simulink model "heave_tracking"  (R2020a)
settings: Solver=VariableStepAuto  StartTime=0.0  StopTime=50  FixedStep=0.001  MaxStep=0.001  RelTol=1e-3  EnableMultiTasking=on
values from neighbouring files (symbols this model uses):
  aw = -728/(1862.87+3660)    (= -0.131815523451)    [heave_tracking_1.m]
  bw = 1/(1862.87+3660)    (= 0.000181065279465)    [heave_tracking_1.m]
  F = [K eye(mm)]*inv(TT)    [heave_tracking_1.m]
  Z_w_bar = -1821/(1862.87+3660)    (= -0.329719873906)    [heave_tracking_1.m]
settings Model: Creator=xiaoran  LastModifiedBy=xiaoran
settings DataIOCC: LimitDataPoints=on  SaveFormat=Array  ReturnWorkspaceOutputs=off
settings OptimizationCC: LifeSpan=inf
settings DebuggingCC: UnderspecifiedInitializationDetection=Classic  MergeDetectMultiDrivingBlocksExec=none  SolverPrmCheckMsg=warning  StateNameClashWarn=warning  SFUnexpectedBacktrackingDiag=warning  SFNoUnconditionalDefaultTransitionDiag=warning  SFExecutionAtInitializationDiag=none  ArithmeticOperatorsInVariantConditions=warning
settings HardwareCC: ProdBitPerPointer=32  ProdBitPerSizeT=32  ProdBitPerPtrDiffT=32  ProdLargestAtomicFloat=None  ProdIntDivRoundTo=Undefined  ProdEndianess=Unspecified  ProdWordSize=32  ProdHWDeviceType=32-bit Generic
settings ModelReferenceCC: PropagateSignalLabelsOutOfModel=off
settings SFSimCC: SimUseLocalCustomCode=off  CustomCodeUndefinedFunction=UseInterfaceOnly
settings RTWCC: RTWUseLocalCustomCode=off
settings CodeAppCC: StateflowObjectComments=on
settings GRTTargetCC: TargetLangStandard=C89/C90 (ANSI)
settings ConfigComp: CovMetricSettings=dw  CovHtmlReporting=on  CovSaveCumulativeToWorkspaceVar=on  CovSaveSingleToWorkspaceVar=on  CovExternalEMLEnable=off

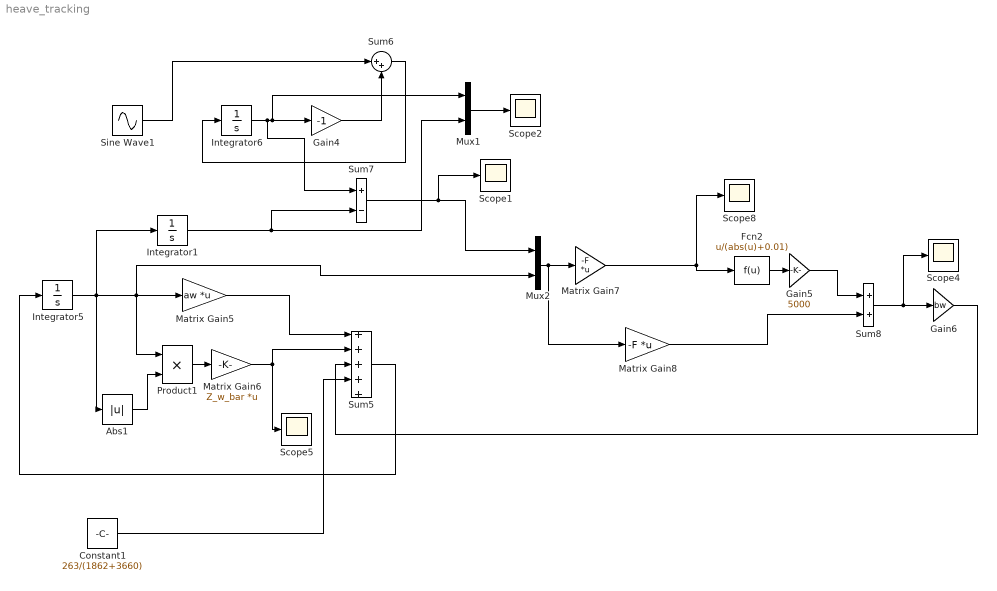
== system heave_tracking ==
  Abs1 : Abs
  Constant1 : Constant  Value=263/(1862+3660)
  Fcn2 : Fcn  Expr=u/(abs(u)+0.01)
  Gain4 : Gain  Gain=-1
  Gain5 : Gain  Gain=5000  SaturateOnIntegerOverflow=on  OutDataTypeStr=Inherit: Same as input  ParamDataTypeStr=Inherit: Same as input
  Gain6 : Gain  Gain=bw  SaturateOnIntegerOverflow=on  OutDataTypeStr=Inherit: Same as input  ParamDataTypeStr=Inherit: Same as input
  Integrator1 : Integrator  InitialCondition=0.1
  Integrator5 : Integrator  InitialCondition=0.1
  Integrator6 : Integrator  InitialCondition=.1
  Matrix Gain5 : Gain  Gain=aw  Multiplication=Matrix(K*u)  SaturateOnIntegerOverflow=on  OutDataTypeStr=Inherit: Same as input  ParamDataTypeStr=Inherit: Same as input
  Matrix Gain6 : Gain  Gain=Z_w_bar  Multiplication=Matrix(K*u)  SaturateOnIntegerOverflow=on  OutDataTypeStr=Inherit: Same as input  ParamDataTypeStr=Inherit: Same as input
  Matrix Gain7 : Gain  Gain=-F  Multiplication=Matrix(K*u)  SaturateOnIntegerOverflow=on  OutDataTypeStr=Inherit: Same as input  ParamDataTypeStr=Inherit: Same as input
  Matrix Gain8 : Gain  Gain=-F  Multiplication=Matrix(K*u)  SaturateOnIntegerOverflow=on  OutDataTypeStr=Inherit: Same as input  ParamDataTypeStr=Inherit: Same as input
  Mux1 : Mux  Inputs=2
  Mux2 : Mux  Inputs=2
  Product1 : Product
  Scope{1..2,4..5,8} (5 alike) : Scope
  Sine Wave1 : Sin  SampleTime=0
  Sum5 : Sum  Inputs=+++++  InputSameDT=on  SaturateOnIntegerOverflow=on  OutDataTypeStr=Inherit: Same as first input
  Sum6 : Sum  Inputs=|++
  Sum7 : Sum  Inputs=+-  InputSameDT=on  SaturateOnIntegerOverflow=on  OutDataTypeStr=Inherit: Same as first input
  Sum8 : Sum  InputSameDT=on  SaturateOnIntegerOverflow=on  OutDataTypeStr=Inherit: Same as first input
  wires:
  Abs1/1 -> Product1/2
  Product1/1 -> Matrix Gain6/1
  Matrix Gain5/1 -> Sum5/1
  Matrix Gain6/1 -> Scope5/1, Sum5/2
  Sum5/1 -> Integrator5/1
  Sum6/1 -> Integrator6/1
  Gain4/1 -> Sum6/2
  Integrator6/1 -> Mux1/1, Gain4/1, Sum7/1
  Integrator5/1 -> Integrator1/1, Abs1/1, Product1/1, Mux2/2, Matrix Gain5/1
  Sum7/1 -> Scope1/1, Mux2/1
  Mux2/1 -> Matrix Gain7/1, Matrix Gain8/1
  Fcn2/1 -> Gain5/1
  Sum8/1 -> Scope4/1, Gain6/1
  Gain6/1 -> Sum5/3
  Mux1/1 -> Scope2/1
  Sine Wave1/1 -> Sum6/1
  Integrator1/1 -> Mux1/2, Sum7/2
  Matrix Gain7/1 -> Fcn2/1, Scope8/1
  Matrix Gain8/1 -> Sum8/2
  Gain5/1 -> Sum8/1
  Constant1/1 -> Sum5/4
